simulink model "DDOSnapad"  (R2018a)
settings: Solver=VariableStepAuto  StartTime=0.0  StopTime=100  RelTol=1e-3
InitFcn:
  | global brojac_normalnih brojac_napadaca;
  | brojac_normalnih = 0;
  | brojac_napadaca = 0;
StartFcn:
  | global brojac_normalnih brojac_napadaca;
  | brojac_normalnih = 0;
  | brojac_napadaca = 0;
undefined symbols (not defined in the file): m, n
settings Model: Creator=User  LastModifiedBy=User

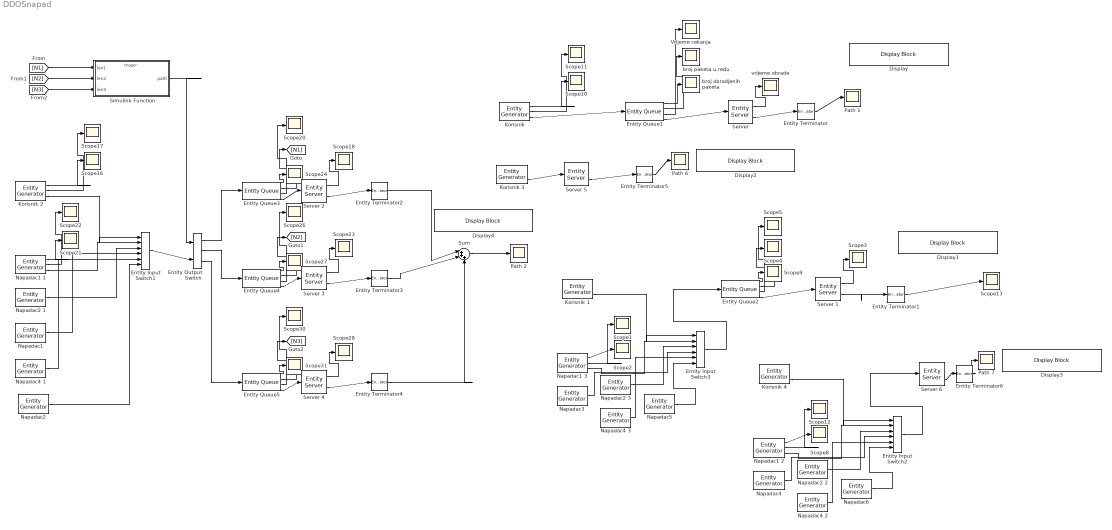
== system DDOSnapad ==
  Display : DisplayBlock  WebBlockId=144  LabelPosition=Hide
  Display1 : DisplayBlock  WebBlockId=257  LabelPosition=Hide
  Display2 : DisplayBlock  WebBlockId=149  LabelPosition=Hide
  Display3 : DisplayBlock  WebBlockId=165  LabelPosition=Hide
  Display4 : DisplayBlock  WebBlockId=260  LabelPosition=Hide
  Entity Input Switch1 : EntityInputSwitch  InputPortMessageModes=m,m,m,m,m,m  OutputPortMessageModes=m  NumberInputPorts=6
      settings: InputPortMap=u1,u2,u3,u4,u5,u6
  Entity Input Switch2 : EntityInputSwitch  InputPortMessageModes=m,m,m,m,m,m  OutputPortMessageModes=m  NumberInputPorts=6
      settings: InputPortMap=u1,u2,u3,u4,u5,u6
  Entity Input Switch3 : EntityInputSwitch  InputPortMessageModes=m,m,m,m,m,m  OutputPortMessageModes=m  NumberInputPorts=6
      settings: InputPortMap=u1,u2,u3,u4,u5,u6
  Entity Output Switch : EntityOutputSwitch  InputPortMessageModes=m,m  OutputPortMessageModes=m,m,m  NumberOutputPorts=3  SwitchingCriterion=From control port  SwitchAttributeName=Attribute1
      settings: InputPortMap=u0,u1  OutputPortMap=o0,o1,o2
  Entity Queue1 : EntityQueue  InputPortMessageModes=m  OutputPortMessageModes=n,n,n,m  Capacity=100  NumberEntitiesDeparted=on  NumberEntitiesInBlock=on  AverageWait=on
      settings: OutputPortMap=o0,o1,o2,o5
  Entity Queue{2..5} (4 alike) : EntityQueue  InputPortMessageModes=m  OutputPortMessageModes=n,n,n,m  Capacity=500  NumberEntitiesDeparted=on  NumberEntitiesInBlock=on  AverageWait=on
      settings: OutputPortMap=o0,o1,o2,o5
  Entity Terminator{,1..6} (7 alike) : EntityTerminator  InputPortMessageModes=m  NumberEntitiesArrived=on
      settings: OutputPortMap=o0
  "Korisnik " : EntityGenerator  OutputPortMessageModes=n,n,m  TimeSource=MATLAB action  IntergenerationTimeAction=|  GenerateAction=|  AttributeName=vrijeme  AttributeInitialValue=0  NumberEntitiesDeparted=on  AverageIntergenerationTime=on  EntityType=Structured  EntityTypeName=vrijeme  DataInitialValue=1
      | persistent rngInit;
      | if isempty(rngInit)
      |     seed = 12345;
      |     rng(seed);
      |     rngInit = true;
      | end
      | 
      | % Pattern: Uniform distribution
      | % m: Minimum, M: Maximum
      | m = 0.1, M = 1;
      | dt = m + (M - m) * rand;
      | persistent rngInit;
      | if isempty(rngInit)
      |     seed = 12345;
      |     rng(seed);
      |     rngInit = true;
      | end
      | 
      | % Pattern: Uniform distribution
      | % m: Minimum, M: Maximum
      | m = 0.1, M = 0.5;
      | entity.vrijeme = m + (M - m) * rand;
      settings: OutputPortMap=o0,o2,o3
  Korisnik 1 : EntityGenerator  OutputPortMessageModes=n,n,m  TimeSource=MATLAB action  IntergenerationTimeAction=|  GenerateAction=|  AttributeName=vrijeme  AttributeInitialValue=0  NumberEntitiesDeparted=on  AverageIntergenerationTime=on  EntityType=Structured  EntityTypeName=vrijeme  DataInitialValue=1
      | persistent rngInit;
      | if isempty(rngInit)
      |     seed = 12345;
      |     rng(seed);
      |     rngInit = true;
      | end
      | 
      | % Pattern: Uniform distribution
      | % m: Minimum, M: Maximum
      | m = 0.1, M = 1;
      | dt = m + (M - m) * rand;
      | persistent rngInit;
      | if isempty(rngInit)
      |     seed = 12345;
      |     rng(seed);
      |     rngInit = true;
      | end
      | 
      | % Pattern: Uniform distribution
      | % m: Minimum, M: Maximum
      | m = 0.1, M = 0.5;
      | entity.vrijeme = m + (M - m) * rand;
      settings: OutputPortMap=o0,o2,o3
  Korisnik 2 : EntityGenerator  OutputPortMessageModes=n,n,m  TimeSource=MATLAB action  IntergenerationTimeAction=|  GenerateAction=|  AttributeName=vrijeme  AttributeInitialValue=0  NumberEntitiesDeparted=on  AverageIntergenerationTime=on  EntityType=Structured  EntityTypeName=vrijeme  DataInitialValue=1
      | persistent rngInit;
      | if isempty(rngInit)
      |     seed = 12345;
      |     rng(seed);
      |     rngInit = true;
      | end
      | 
      | % Pattern: Uniform distribution
      | % m: Minimum, M: Maximum
      | m = 0.1, M = 2;
      | dt = m + (M - m) * rand;
      | persistent rngInit;
      | if isempty(rngInit)
      |     seed = 12345;
      |     rng(seed);
      |     rngInit = true;
      | end
      | computeRouting();
      | % Pattern: Uniform distribution
      | % m: Minimum, M: Maximum
      | m = 0.1, M = 0.5;
      | entity.vrijeme = m + (M - m) * rand;
      settings: OutputPortMap=o0,o2,o3
  Korisnik 3 : EntityGenerator  OutputPortMessageModes=n,n,m  TimeSource=MATLAB action  IntergenerationTimeAction=|  GenerateAction=|  AttributeName=vrijeme  AttributeInitialValue=0  NumberEntitiesDeparted=on  AverageIntergenerationTime=on  EntityType=Structured  EntityTypeName=vrijeme  DataInitialValue=1
      | persistent rngInit;
      | if isempty(rngInit)
      |     seed = 12345;
      |     rng(seed);
      |     rngInit = true;
      | end
      | 
      | % Pattern: Uniform distribution
      | % m: Minimum, M: Maximum
      | m = 0.1, M = 1;
      | dt = m + (M - m) * rand;
      | persistent rngInit;
      | if isempty(rngInit)
      |     seed = 12345;
      |     rng(seed);
      |     rngInit = true;
      | end
      | 
      | % Pattern: Uniform distribution
      | % m: Minimum, M: Maximum
      | m = 0.1, M = 0.5;
      | entity.vrijeme = m + (M - m) * rand;
      settings: OutputPortMap=o0,o2,o3
  Korisnik 4 : EntityGenerator  OutputPortMessageModes=n,n,m  TimeSource=MATLAB action  IntergenerationTimeAction=|  GenerateAction=|  AttributeName=vrijeme  AttributeInitialValue=0  NumberEntitiesDeparted=on  AverageIntergenerationTime=on  EntityType=Structured  EntityTypeName=vrijeme  DataInitialValue=1
      | persistent rngInit;
      | if isempty(rngInit)
      |     seed = 12345;
      |     rng(seed);
      |     rngInit = true;
      | end
      | 
      | % Pattern: Uniform distribution
      | % m: Minimum, M: Maximum
      | m = 0.1, M = 2;
      | dt = m + (M - m) * rand;
      | persistent rngInit;
      | if isempty(rngInit)
      |     seed = 12345;
      |     rng(seed);
      |     rngInit = true;
      | end
      | 
      | % Pattern: Uniform distribution
      | % m: Minimum, M: Maximum
      | m = 0.1, M = 1;
      | entity.vrijeme = m + (M - m) * rand;
      settings: OutputPortMap=o0,o2,o3
  Napadac1 : EntityGenerator  OutputPortMessageModes=m  TimeSource=MATLAB action  IntergenerationTimeAction=|  GenerateAction=|  AttributeName=vrijeme  AttributeInitialValue=0  EntityType=Structured  EntityTypeName=vrijeme  DataInitialValue=1
      | persistent rngInit;
      | if isempty(rngInit)
      |     seed = 12345;
      |     rng(seed);
      |     rngInit = true;
      | end
      | 
      | % Pattern: Uniform distribution
      | % m: Minimum, M: Maximum
      | m = 0.005, M = 0.02;
      | dt = m + (M - m) * rand;
      | computeRouting();
      | persistent rngInit;
      | if isempty(rngInit)
      |     seed = 12345;
      |     rng(seed);
      |     rngInit = true;
      | end
      | 
      | % Pattern: Uniform distribution
      | % m: Minimum, M: Maximum
      | m = 0.005, M = 0.02;
      | entity.vrijeme = m + (M - m) * rand;
  Napadac1 1 : EntityGenerator  OutputPortMessageModes=n,n,m  TimeSource=MATLAB action  IntergenerationTimeAction=|  GenerateAction=|  AttributeName=vrijeme  AttributeInitialValue=0  NumberEntitiesDeparted=on  AverageIntergenerationTime=on  EntityType=Structured  EntityTypeName=vrijeme  DataInitialValue=1
      | persistent rngInit;
      | if isempty(rngInit)
      |     seed = 12345;
      |     rng(seed);
      |     rngInit = true;
      | end
      | 
      | % Pattern: Uniform distribution
      | % m: Minimum, M: Maximum
      | m = 0.005, M = 0.02;
      | dt = m + (M - m) * rand;
      | persistent rngInit;
      | if isempty(rngInit)
      |     seed = 12345;
      |     rng(seed);
      |     rngInit = true;
      | end
      | computeRouting();
      | % Pattern: Uniform distribution
      | % m: Minimum, M: Maximum
      | m = 0.005, M = 0.02;
      | entity.vrijeme = m + (M - m) * rand;
      settings: OutputPortMap=o0,o2,o3
  Napadac1 2 : EntityGenerator  OutputPortMessageModes=n,n,m  TimeSource=MATLAB action  IntergenerationTimeAction=|  GenerateAction=|  AttributeName=vrijeme  AttributeInitialValue=0  NumberEntitiesDeparted=on  AverageIntergenerationTime=on  EntityType=Structured  EntityTypeName=vrijeme  DataInitialValue=1
      | persistent rngInit;
      | if isempty(rngInit)
      |     seed = 12345;
      |     rng(seed);
      |     rngInit = true;
      | end
      | 
      | % Pattern: Uniform distribution
      | % m: Minimum, M: Maximum
      | m = 0.005, M = 0.02;
      | dt = m + (M - m) * rand;
      | persistent rngInit;
      | if isempty(rngInit)
      |     seed = 12345;
      |     rng(seed);
      |     rngInit = true;
      | end
      | 
      | % Pattern: Uniform distribution
      | % m: Minimum, M: Maximum
      | m = 0.005, M = 0.02;
      | entity.vrijeme = m + (M - m) * rand;
      settings: OutputPortMap=o0,o2,o3
  Napadac1 3 : EntityGenerator  OutputPortMessageModes=n,n,m  TimeSource=MATLAB action  IntergenerationTimeAction=|  GenerateAction=|  AttributeName=vrijeme  AttributeInitialValue=0  NumberEntitiesDeparted=on  AverageIntergenerationTime=on  EntityType=Structured  EntityTypeName=vrijeme  DataInitialValue=1
      | persistent rngInit;
      | if isempty(rngInit)
      |     seed = 12345;
      |     rng(seed);
      |     rngInit = true;
      | end
      | 
      | % Pattern: Uniform distribution
      | % m: Minimum, M: Maximum
      | m = 0.005, M = 0.02;
      | dt = m + (M - m) * rand;
      | persistent rngInit;
      | if isempty(rngInit)
      |     seed = 12345;
      |     rng(seed);
      |     rngInit = true;
      | end
      | 
      | % Pattern: Uniform distribution
      | % m: Minimum, M: Maximum
      | m = 0.005, M = 0.02;
      | entity.vrijeme = m + (M - m) * rand;
      settings: OutputPortMap=o0,o2,o3
  Napadac2 : EntityGenerator  OutputPortMessageModes=m  TimeSource=MATLAB action  IntergenerationTimeAction=|  GenerateAction=|  AttributeName=vrijeme  AttributeInitialValue=0  EntityType=Structured  EntityTypeName=vrijeme  DataInitialValue=1
      | persistent rngInit;
      | if isempty(rngInit)
      |     seed = 12345;
      |     rng(seed);
      |     rngInit = true;
      | end
      | 
      | % Pattern: Uniform distribution
      | % m: Minimum, M: Maximum
      | m = 0.005, M = 0.02;
      | dt = m + (M - m) * rand;
      | computeRouting();
      | persistent rngInit;
      | if isempty(rngInit)
      |     seed = 12345;
      |     rng(seed);
      |     rngInit = true;
      | end
      | 
      | % Pattern: Uniform distribution
      | % m: Minimum, M: Maximum
      | m = 0.005, M = 0.02;
      | entity.vrijeme = m + (M - m) * rand;
  Napadac2 1 : EntityGenerator  OutputPortMessageModes=m  TimeSource=MATLAB action  IntergenerationTimeAction=|  GenerateAction=|  AttributeName=vrijeme  AttributeInitialValue=0  EntityType=Structured  EntityTypeName=vrijeme  DataInitialValue=1
      | persistent rngInit;
      | if isempty(rngInit)
      |     seed = 12345;
      |     rng(seed);
      |     rngInit = true;
      | end
      | 
      | % Pattern: Uniform distribution
      | % m: Minimum, M: Maximum
      | m = 0.005, M = 0.02;
      | dt = m + (M - m) * rand;
      | computeRouting();
      | persistent rngInit;
      | if isempty(rngInit)
      |     seed = 12345;
      |     rng(seed);
      |     rngInit = true;
      | end
      | 
      | % Pattern: Uniform distribution
      | % m: Minimum, M: Maximum
      | m = 0.005, M = 0.02;
      | entity.vrijeme = m + (M - m) * rand;
  Napadac2 2 : EntityGenerator  OutputPortMessageModes=m  TimeSource=MATLAB action  IntergenerationTimeAction=|  GenerateAction=|  AttributeName=vrijeme  AttributeInitialValue=0  EntityType=Structured  EntityTypeName=vrijeme  DataInitialValue=1
      | persistent rngInit;
      | if isempty(rngInit)
      |     seed = 12345;
      |     rng(seed);
      |     rngInit = true;
      | end
      | 
      | % Pattern: Uniform distribution
      | % m: Minimum, M: Maximum
      | m = 0.005, M = 0.02;
      | dt = m + (M - m) * rand;
      | persistent rngInit;
      | if isempty(rngInit)
      |     seed = 12345;
      |     rng(seed);
      |     rngInit = true;
      | end
      | 
      | % Pattern: Uniform distribution
      | % m: Minimum, M: Maximum
      | m = 0.005, M = 0.02;
      | entity.vrijeme = m + (M - m) * rand;
  Napadac2 3 : EntityGenerator  OutputPortMessageModes=m  TimeSource=MATLAB action  IntergenerationTimeAction=|  GenerateAction=|  AttributeName=vrijeme  AttributeInitialValue=0  EntityType=Structured  EntityTypeName=vrijeme  DataInitialValue=1
      | persistent rngInit;
      | if isempty(rngInit)
      |     seed = 12345;
      |     rng(seed);
      |     rngInit = true;
      | end
      | 
      | % Pattern: Uniform distribution
      | % m: Minimum, M: Maximum
      | m = 0.005, M = 0.02;
      | dt = m + (M - m) * rand;
      | persistent rngInit;
      | if isempty(rngInit)
      |     seed = 12345;
      |     rng(seed);
      |     rngInit = true;
      | end
      | 
      | % Pattern: Uniform distribution
      | % m: Minimum, M: Maximum
      | m = 0.005, M = 0.02;
      | entity.vrijeme = m + (M - m) * rand;
  Napadac3 : EntityGenerator  OutputPortMessageModes=m  TimeSource=MATLAB action  IntergenerationTimeAction=|  GenerateAction=|  AttributeName=vrijeme  AttributeInitialValue=0  EntityType=Structured  EntityTypeName=vrijeme  DataInitialValue=1
      | persistent rngInit;
      | if isempty(rngInit)
      |     seed = 12345;
      |     rng(seed);
      |     rngInit = true;
      | end
      | 
      | % Pattern: Uniform distribution
      | % m: Minimum, M: Maximum
      | m = 0.005, M = 0.02;
      | dt = m + (M - m) * rand;
      | persistent rngInit;
      | if isempty(rngInit)
      |     seed = 12345;
      |     rng(seed);
      |     rngInit = true;
      | end
      | 
      | % Pattern: Uniform distribution
      | % m: Minimum, M: Maximum
      | m = 0.005, M = 0.02;
      | entity.vrijeme = m + (M - m) * rand;
  Napadac4 : EntityGenerator  OutputPortMessageModes=m  TimeSource=MATLAB action  IntergenerationTimeAction=|  GenerateAction=|  AttributeName=vrijeme  AttributeInitialValue=0  EntityType=Structured  EntityTypeName=vrijeme  DataInitialValue=1
      | persistent rngInit;
      | if isempty(rngInit)
      |     seed = 12345;
      |     rng(seed);
      |     rngInit = true;
      | end
      | 
      | % Pattern: Uniform distribution
      | % m: Minimum, M: Maximum
      | m = 0.005, M = 0.02;
      | dt = m + (M - m) * rand;
      | persistent rngInit;
      | if isempty(rngInit)
      |     seed = 12345;
      |     rng(seed);
      |     rngInit = true;
      | end
      | 
      | % Pattern: Uniform distribution
      | % m: Minimum, M: Maximum
      | m = 0.005, M = 0.02;
      | entity.vrijeme = m + (M - m) * rand;
  Napadac4 1 : EntityGenerator  OutputPortMessageModes=m  TimeSource=MATLAB action  IntergenerationTimeAction=|  GenerateAction=|  AttributeName=vrijeme  AttributeInitialValue=0  EntityType=Structured  EntityTypeName=vrijeme  DataInitialValue=1
      | persistent rngInit;
      | if isempty(rngInit)
      |     seed = 12345;
      |     rng(seed);
      |     rngInit = true;
      | end
      | 
      | % Pattern: Uniform distribution
      | % m: Minimum, M: Maximum
      | m = 0.005, M = 0.02;
      | dt = m + (M - m) * rand;
      | computeRouting();
      | persistent rngInit;
      | if isempty(rngInit)
      |     seed = 12345;
      |     rng(seed);
      |     rngInit = true;
      | end
      | 
      | % Pattern: Uniform distribution
      | % m: Minimum, M: Maximum
      | m = 0.005, M = 0.02;
      | entity.vrijeme = m + (M - m) * rand;
  Napadac4 2 : EntityGenerator  OutputPortMessageModes=m  TimeSource=MATLAB action  IntergenerationTimeAction=|  GenerateAction=|  AttributeName=vrijeme  AttributeInitialValue=0  EntityType=Structured  EntityTypeName=vrijeme  DataInitialValue=1
      | persistent rngInit;
      | if isempty(rngInit)
      |     seed = 12345;
      |     rng(seed);
      |     rngInit = true;
      | end
      | 
      | % Pattern: Uniform distribution
      | % m: Minimum, M: Maximum
      | m = 0.005, M = 0.02;
      | dt = m + (M - m) * rand;
      | persistent rngInit;
      | if isempty(rngInit)
      |     seed = 12345;
      |     rng(seed);
      |     rngInit = true;
      | end
      | 
      | % Pattern: Uniform distribution
      | % m: Minimum, M: Maximum
      | m = 0.005, M = 0.02;
      | entity.vrijeme = m + (M - m) * rand;
  Napadac4 3 : EntityGenerator  OutputPortMessageModes=m  TimeSource=MATLAB action  IntergenerationTimeAction=|  GenerateAction=|  AttributeName=vrijeme  AttributeInitialValue=0  EntityType=Structured  EntityTypeName=vrijeme  DataInitialValue=1
      | persistent rngInit;
      | if isempty(rngInit)
      |     seed = 12345;
      |     rng(seed);
      |     rngInit = true;
      | end
      | 
      | % Pattern: Uniform distribution
      | % m: Minimum, M: Maximum
      | m = 0.005, M = 0.02;
      | dt = m + (M - m) * rand;
      | persistent rngInit;
      | if isempty(rngInit)
      |     seed = 12345;
      |     rng(seed);
      |     rngInit = true;
      | end
      | 
      | % Pattern: Uniform distribution
      | % m: Minimum, M: Maximum
      | m = 0.005, M = 0.02;
      | entity.vrijeme = m + (M - m) * rand;
  Napadac5 : EntityGenerator  OutputPortMessageModes=m  TimeSource=MATLAB action  IntergenerationTimeAction=|  GenerateAction=|  AttributeName=vrijeme  AttributeInitialValue=0  EntityType=Structured  EntityTypeName=vrijeme  DataInitialValue=1
      | persistent rngInit;
      | if isempty(rngInit)
      |     seed = 12345;
      |     rng(seed);
      |     rngInit = true;
      | end
      | 
      | % Pattern: Uniform distribution
      | % m: Minimum, M: Maximum
      | m = 0.005, M = 0.02;
      | dt = m + (M - m) * rand;
      | persistent rngInit;
      | if isempty(rngInit)
      |     seed = 12345;
      |     rng(seed);
      |     rngInit = true;
      | end
      | 
      | % Pattern: Uniform distribution
      | % m: Minimum, M: Maximum
      | m = 0.005, M = 0.02;
      | entity.vrijeme = m + (M - m) * rand;
  Napadac6 : EntityGenerator  OutputPortMessageModes=m  TimeSource=MATLAB action  IntergenerationTimeAction=|  GenerateAction=|  AttributeName=vrijeme  AttributeInitialValue=0  EntityType=Structured  EntityTypeName=vrijeme  DataInitialValue=1
      | persistent rngInit;
      | if isempty(rngInit)
      |     seed = 12345;
      |     rng(seed);
      |     rngInit = true;
      | end
      | 
      | % Pattern: Uniform distribution
      | % m: Minimum, M: Maximum
      | m = 0.005, M = 0.02;
      | dt = m + (M - m) * rand;
      | persistent rngInit;
      | if isempty(rngInit)
      |     seed = 12345;
      |     rng(seed);
      |     rngInit = true;
      | end
      | 
      | % Pattern: Uniform distribution
      | % m: Minimum, M: Maximum
      | m = 0.005, M = 0.02;
      | entity.vrijeme = m + (M - m) * rand;
  Path {1..2,6..7} (4 alike) : Scope
  Scope{1..5,8..13,16..18,20..24,26..28,30..31} (24 alike) : Scope
  "Server " : EntityServer  InputPortMessageModes=m  OutputPortMessageModes=n,m  Capacity=2  ServiceTimeSource=Attribute  ServiceTimeAttributeName=vrijeme  Utilization=on
      settings: OutputPortMap=o5,o9
  Server {1..4} (4 alike) : EntityServer  InputPortMessageModes=m  OutputPortMessageModes=n,m  Capacity=4  ServiceTimeSource=Attribute  ServiceTimeAttributeName=vrijeme  Utilization=on
      settings: OutputPortMap=o5,o9
  Server 5 : EntityServer  InputPortMessageModes=m  OutputPortMessageModes=n,m  Capacity=inf  ServiceTimeSource=Attribute  ServiceTimeAttributeName=vrijeme  Utilization=on
      settings: OutputPortMap=o5,o9
  Server 6 : EntityServer  InputPortMessageModes=m  OutputPortMessageModes=n,m  Capacity=inf  ServiceTimeSource=Attribute  ServiceTimeAttributeName=vrijeme  Utilization=on
      settings: OutputPortMap=o5,o9
  Simulink Function : Subsystem  TreatAsAtomicUnit=on
  Sum : Sum  Inputs=|+++
  Vrijeme cekanja : Scope
  broj obradjenih paketa : Scope
  "broj paketa u redu " : Scope
  "vrijeme obrade " : Scope
  wires:
  "Korisnik "/3 -> Entity Queue1/1
  Entity Queue1/3 -> Vrijeme cekanja/1
  Entity Queue1/2 -> "broj paketa u redu "/1
  Entity Queue1/4 -> "Server "/1
  "Korisnik "/1 -> Scope10/1
  "Server "/1 -> "vrijeme obrade "/1
  "Korisnik "/2 -> Scope11/1
  "Server "/2 -> Entity Terminator/1
  Entity Terminator/1 -> Path 1/1
  Entity Queue2/4 -> Server 1/1
  Entity Queue2/3 -> Scope5/1
  Entity Queue2/2 -> Scope4/1
  Server 1/1 -> Scope3/1
  Entity Queue2/1 -> Scope9/1
  Entity Queue1/1 -> broj obradjenih paketa/1
  Korisnik 2/3 -> Entity Input Switch1/1
  Entity Queue3/1 -> Scope24/1
  Napadac1 1/2 -> Scope22/1
  Napadac4 1/1 -> Entity Input Switch1/5
  Napadac2 1/1 -> Entity Input Switch1/3
  Entity Queue3/2 -> [N1]
  Server 2/2 -> Entity Terminator2/1
  Korisnik 2/2 -> Scope17/1
  Server 2/1 -> Scope18/1
  Korisnik 2/1 -> Scope16/1
  Entity Queue3/3 -> Scope20/1
  Napadac1 1/1 -> Scope21/1
  Napadac1 1/3 -> Entity Input Switch1/2
  Entity Terminator2/1 -> Sum/1
  Napadac2/1 -> Entity Input Switch1/6
  Napadac1/1 -> Entity Input Switch1/4
  Entity Queue3/4 -> Server 2/1
  Entity Input Switch1/1 -> Entity Output Switch/2
  Entity Output Switch/1 -> Entity Queue3/1
  Server 3/1 -> Scope23/1
  Entity Queue4/3 -> Scope26/1
  Entity Queue4/4 -> Server 3/1
  Server 3/2 -> Entity Terminator3/1
  Entity Queue4/2 -> [N2]
  Entity Terminator3/1 -> Sum/2
  Entity Queue4/1 -> Scope27/1
  Server 4/1 -> Scope28/1
  Entity Queue5/3 -> Scope30/1
  Entity Queue5/4 -> Server 4/1
  Server 4/2 -> Entity Terminator4/1
  Entity Queue5/2 -> [N3]
  Entity Terminator4/1 -> Sum/3
  Entity Queue5/1 -> Scope31/1
  Entity Output Switch/2 -> Entity Queue4/1
  Entity Output Switch/3 -> Entity Queue5/1
  [N1] -> Simulink Function/1(len1)
  [N2] -> Simulink Function/2(len2)
  Simulink Function/1(path) -> Entity Output Switch/1
  [N3] -> Simulink Function/3(len3)
  Korisnik 3/3 -> Server 5/1
  Server 5/2 -> Entity Terminator5/1
  Entity Terminator5/1 -> Path 6/1
  Korisnik 4/3 -> Entity Input Switch2/1
  Napadac2 2/1 -> Entity Input Switch2/3
  Napadac4 2/1 -> Entity Input Switch2/5
  Entity Input Switch2/1 -> Server 6/1
  Napadac6/1 -> Entity Input Switch2/6
  Napadac1 2/2 -> Scope12/1
  Napadac4/1 -> Entity Input Switch2/4
  Napadac1 2/3 -> Entity Input Switch2/2
  Napadac1 2/1 -> Scope8/1
  Server 6/2 -> Entity Terminator6/1
  Entity Terminator6/1 -> Path 7/1
  Server 1/2 -> Entity Terminator1/1
  Entity Terminator1/1 -> Scope13/1
  Napadac1 3/2 -> Scope1/1
  Napadac3/1 -> Entity Input Switch3/4
  Napadac2 3/1 -> Entity Input Switch3/3
  Napadac4 3/1 -> Entity Input Switch3/5
  Napadac5/1 -> Entity Input Switch3/6
  Napadac1 3/1 -> Scope2/1
  Entity Input Switch3/1 -> Entity Queue2/1
  Korisnik 1/3 -> Entity Input Switch3/1
  Napadac1 3/3 -> Entity Input Switch3/2
  Sum/1 -> Path 2/1

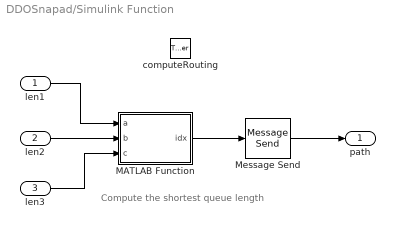
== system DDOSnapad/Simulink Function ==
  note: Compute the shortest queue length
  len1 : Inport
  len2 : Inport  Port=2
  len3 : Inport  Port=3
  computeRouting : TriggerPort  TriggerType=function-call  IsSimulinkFunction=on  FunctionName=computeRouting  VariantControl=Variant
  MATLAB Function : MATLAB Function  TreatAsAtomicUnit=on
  Message Send : MessageSend  OutputPortMessageModes=m
      settings: InputPortMap=u1
  path : Outport
  wires:
  len1/1 -> MATLAB Function/1(a)
  len2/1 -> MATLAB Function/2(b)
  len3/1 -> MATLAB Function/3(c)
  MATLAB Function/1(idx) -> Message Send/1
  Message Send/1 -> path/1

== matlab function DDOSnapad/Simulink Function/MATLAB Function ==
  data: a input; idx output; b input; c input
function idx = fcn(a,b,c)

[~, idx] = min([a,b,c]);
